simulink model "Trim_Pioneer"  (R2018a)
settings: Solver=VariableStepAuto  StartTime=0.0  StopTime=30  RelTol=1e-3  EnableMultiTasking=on
libraries: airlib x1
settings Model: Creator=MONCAYOH  LastModifiedBy=enriqueg
settings DataIOCC: SaveFormat=Array  SignalLoggingSaveFormat=ModelDataLogs  SaveOutput=off  SaveTime=off
settings OptimizationCC: BlockReduction=off  BooleanDataType=off
settings DebuggingCC: SaveWithParameterizedLinksMsg=none  UnderspecifiedInitializationDetection=Classic  MergeDetectMultiDrivingBlocksExec=none  SignalResolutionControl=TryResolveAllWithWarning  MultiTaskDSMMsg=warning  MultiTaskCondExecSysMsg=none
settings HardwareCC: TargetUnknown=on
settings ModelReferenceCC: PropagateSignalLabelsOutOfModel=off
settings CodeAppCC: StateflowObjectComments=on
settings GRTTargetCC: TargetLangStandard=C89/C90 (ANSI)  CombineOutputUpdateFcns=off  GRTInterface=on

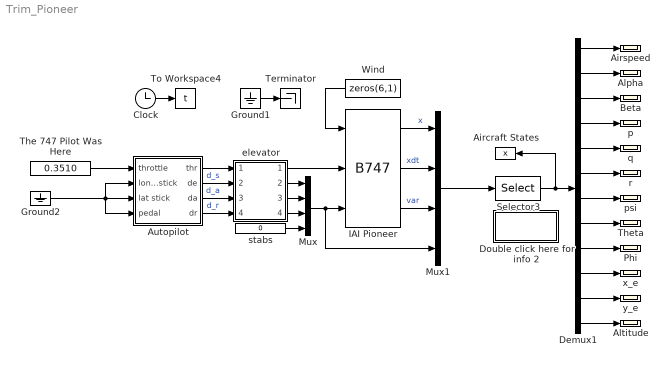
== system Trim_Pioneer ==
  " IAI Pioneer " : airlib/B747  GM1="[0.5486  5.1511  2.8261   47.2259  90.9483  111.4754   0  -6.6462  0   190.512]"  CD_wind="[0.060  0.430  0  0.0180  0]"  CL_wind="[0.385  4.78  8.05  0.401  0]"  Cm_body="[0.194  -2.12   -36.6   -1.76    0]"  CY_body="[0   -0.819    0     0    0.191    0]"  Cl_body="[0   -0.023   -0.450   0.265   -0.161  -0.00229]"  Cn_body="[0    0.109  -0.110  -0.200    0.0200  -0.0917]"  x0="[33.4389 0.1247 0   0 0 0   0 0.1247 0   0 0 150]"
  Aircraft States : ToWorkspace  VariableName=x  SampleTime=0.05
  Airspeed : Scope
  Alpha : Scope
  Altitude : Scope
  Autopilot : Subsystem
  Beta : Scope
  Clock : Clock
  Demux1 : Demux  Outputs=12
  Double click here for info 2 : Subsystem
      mask Display: disp('Output\nSignals')
  Ground1 : Ground
  Ground2 : Ground
  Mux : Mux
  Mux1 : Mux  Inputs=[12 12 12 4]
  Phi : Scope
  Selector3 : Selector  InputPortWidth=40  IndexOptions=Index vector (dialog)  Indices=1:12  OutputSizes=1
  Terminator : Terminator
  The 747 Pilot Was Here : Constant  Value=0.3510
  Theta : Scope
  To Workspace4 : ToWorkspace  VariableName=t  SampleTime=0.05
  Wind : Constant  Value=zeros(6,1)
  elevator : Subsystem
      mask Display: disp('Cable &\nactuator\ndynamics')
  p : Scope
  psi : Scope
  q : Scope
  r : Scope
  stabs : Constant  Value=0
  x_e : Scope
  y_e : Scope
  wires:
  elevator/3(deltaa) -> Mux/2
  elevator/4(deltar) -> Mux/3
  elevator/2(deltae) -> Mux/1
  Autopilot/2(de) -> elevator/2(D_elv)  "d_s"
  Autopilot/3(da) -> elevator/3(D_ail)  "d_a"
  Autopilot/4(dr) -> elevator/4(D_rud)  "d_r"
  Mux/1 -> " IAI Pioneer "/3, Mux1/4
  elevator/1(throttle) -> " IAI Pioneer "/2
  Mux1/1 -> Selector3/1
  Selector3/1 -> Demux1/1, Aircraft States/1
  Demux1/1 -> Airspeed/1
  Demux1/2 -> Alpha/1
  Demux1/3 -> Beta/1
  Demux1/4 -> p/1
  Demux1/5 -> q/1
  Demux1/6 -> r/1
  Demux1/7 -> psi/1
  Demux1/8 -> Theta/1
  Demux1/9 -> Phi/1
  Demux1/10 -> x_e/1
  Demux1/11 -> y_e/1
  Demux1/12 -> Altitude/1
  Autopilot/1(thr) -> elevator/1(D_thr)
  Clock/1 -> To Workspace4/1
  stabs/1 -> Mux/4
  Wind/1 -> " IAI Pioneer "/1
  " IAI Pioneer "/1 -> Mux1/1  "x"
  " IAI Pioneer "/2 -> Mux1/2  "xdt"
  " IAI Pioneer "/3 -> Mux1/3  "var"
  The 747 Pilot Was Here/1 -> Autopilot/1(throttle)
  Ground1/1 -> Terminator/1
  Ground2/1 -> Autopilot/4(pedal), Autopilot/3(lat stick), Autopilot/2(long stick)

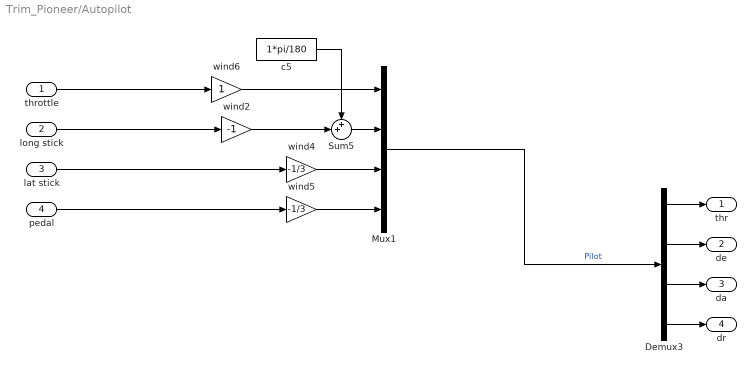
== system Trim_Pioneer/Autopilot ==
  throttle : Inport
  long stick : Inport  Port=2
  lat stick : Inport  Port=3
  pedal : Inport  Port=4
  Demux3 : Demux
  Mux1 : Mux
  Sum5 : Sum  Inputs=++|  SaturateOnIntegerOverflow=on  InputSameDT=on  OutDataTypeStr=Inherit: Same as first input
  c5 : Constant  Value=1*pi/180
  wind2 : Gain  Gain=-1  SaturateOnIntegerOverflow=on  OutDataTypeStr=Inherit: Same as input  ParamDataTypeStr=Inherit: Same as input
  wind4 : Gain  Gain=-1/3  SaturateOnIntegerOverflow=on  OutDataTypeStr=Inherit: Same as input  ParamDataTypeStr=Inherit: Same as input
  wind5 : Gain  Gain=-1/3  SaturateOnIntegerOverflow=on  OutDataTypeStr=Inherit: Same as input  ParamDataTypeStr=Inherit: Same as input
  wind6 : Gain  SaturateOnIntegerOverflow=on  OutDataTypeStr=Inherit: Same as input  ParamDataTypeStr=Inherit: Same as input
  thr : Outport
  de : Outport  Port=2
  da : Outport  Port=3
  dr : Outport  Port=4
  wires:
  long stick/1 -> wind2/1
  lat stick/1 -> wind4/1
  pedal/1 -> wind5/1
  Mux1/1 -> Demux3/1  "Pilot"
  Demux3/1 -> thr/1
  Demux3/2 -> de/1
  Demux3/3 -> da/1
  Demux3/4 -> dr/1
  wind4/1 -> Mux1/3
  wind5/1 -> Mux1/4
  throttle/1 -> wind6/1
  c5/1 -> Sum5/1
  Sum5/1 -> Mux1/2
  wind2/1 -> Sum5/2
  wind6/1 -> Mux1/1

== system Trim_Pioneer/Double click here for info 2 ==
  note: 01 v (m/s)
      | 02 alpha (rad)
      | 03 beta (rad)
      | 04 p (rad/s)
      | 05 q (rad/s)
      | 06 r  (rad/s)
      | 07 psi (rad)
      | 08 theta (rad)
      | 09 phi (rad)
      | 10 xe (m)
      | 11 ye (m)
      | 12 ze (m)
      | 13 v dot (m/s2)
      | 14 alpha dot (rad/s)
      | 15 beta dot (rad/s)
      | 16 p dot (rad/s2)
      | 17 q dot (rad/s2)
      | 18 r dot (rad/s2)
      | 19 fi dot (rad/s)
      | 20 theta dot (rad/s)
      | 21 psi dot (rad/s)
      | 22 xe dot (m/s)
      | 23 ye dot (m/s)
      | 24 ze dot (m/s)
      | 25 u dot (m/s2)
      | 26 v dot (m/s2)
      | 27 w dot (m/s2)
      | 28 pb/2v (rad)
      | 29 qc/v (rad)
      | 30 rb/v (rad)
      | 31 Ax (g)
      | 32 Ay (g)
      | 33 Az (g)
      | 34 ax (g)
      | 35 ay (g)
      | 36 az (g)
      | 37 delta elevators (rad)
      | 38 delta ailerons (rad)
      | 39 delta rudder (rad)
      | 40 delta stabs (rad)

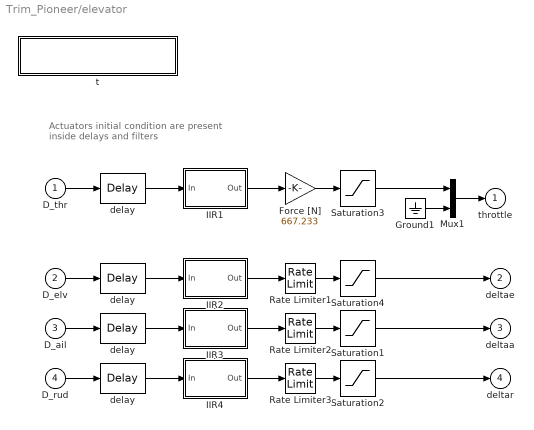
== system Trim_Pioneer/elevator ==
  note: Actuators initial condition are present
      | inside delays and filters
  D_thr : Inport
  D_elv : Inport  Port=2
  D_ail : Inport  Port=3
  D_rud : Inport  Port=4
  " delay" : TransportDelay  DelayTime=0.03  InitialOutput=-1.71374e-004
  " delay " : TransportDelay  DelayTime=0.03  InitialOutput=0.490154
  Force [N] : Gain  Gain=667.233  SaturateOnIntegerOverflow=on  OutDataTypeStr=Inherit: Same as input  ParamDataTypeStr=Inherit: Same as input
  Ground1 : Ground
  IIR1 : Subsystem  mask(Discrete Time First Order IIR){ni=1, a=4, x0=0.490154, T=0.05}
      mask prompts: ni "Number of Channels"; a "Cutoff Frequency (a)"; x0 "Initial Condition"; T "Sample Time"
      mask help:
      | Each channel has the transfer function
      |   (1-exp(-aT))/(1-exp(-aT)(z^-1)) which is a good
      |   (pz-matched) approximation of a/(s+a) if 10*a*T<pi
      mask init:
      | A=[];B=[];C=[];D=[];
      | for i=1:ni,
      | A=[A,zeros(size(A,1),1);zeros(1,size(A,2)),exp(-a*T)];
      | B=[B,zeros(size(B,1),1);zeros(1,size(B,2)),1-exp(-a*T)];
      | C=[C,zeros(size(C,1),1);zeros(1,size(C,2)),exp(-a*T)];
      | D=[D,zeros(size(D,1),1);zeros(1,size(D,2)),1-exp(-a*T)];
      | end
      mask Help:
      | <p>
      |   Each channel has the transfer function
      |   (1-exp(-aT))/(1-exp(-aT)(z^-1)) which is a good
      |   (pz-matched) approximation of a/(s+a) if 10*a*T<pi
      | </p>
      mask Display: dpoly(a,[1 a],'s')
  IIR2 : Subsystem  mask(Discrete Time First Order IIR){ni=1, a=15, x0=-1.71374e-004, T=0.05}
      mask prompts: ni "Number of Channels"; a "Cutoff Frequency (a)"; x0 "Initial Condition"; T "Sample Time"
      mask help:
      | Each channel has the transfer function
      |   (1-exp(-aT))/(1-exp(-aT)(z^-1)) which is a good
      |   (pz-matched) approximation of a/(s+a) if 10*a*T<pi
      mask init: same as Trim_Pioneer/elevator/IIR1
      mask Help:
      | <p>
      |   Each channel has the transfer function
      |   (1-exp(-aT))/(1-exp(-aT)(z^-1)) which is a good
      |   (pz-matched) approximation of a/(s+a) if 10*a*T<pi
      | </p>
      mask Display: dpoly(a,[1 a],'s')
  IIR3 : Subsystem  mask(Discrete Time First Order IIR){ni=1, a=40, x0=0, T=0.05}
      mask prompts: ni "Number of Channels"; a "Cutoff Frequency (a)"; x0 "Initial Condition"; T "Sample Time"
      mask help:
      | Each channel has the transfer function
      |   (1-exp(-aT))/(1-exp(-aT)(z^-1)) which is a good
      |   (pz-matched) approximation of a/(s+a) if 10*a*T<pi
      mask init: same as Trim_Pioneer/elevator/IIR1
      mask Help:
      | <p>
      |   Each channel has the transfer function
      |   (1-exp(-aT))/(1-exp(-aT)(z^-1)) which is a good
      |   (pz-matched) approximation of a/(s+a) if 10*a*T<pi
      | </p>
      mask Display: dpoly(a,[1 a],'s')
  IIR4 : Subsystem  mask(Discrete Time First Order IIR){ni=1, a=15, x0=0, T=0.05}
      mask prompts: ni "Number of Channels"; a "Cutoff Frequency (a)"; x0 "Initial Condition"; T "Sample Time"
      mask help:
      | Each channel has the transfer function
      |   (1-exp(-aT))/(1-exp(-aT)(z^-1)) which is a good
      |   (pz-matched) approximation of a/(s+a) if 10*a*T<pi
      mask init: same as Trim_Pioneer/elevator/IIR1
      mask Help:
      | <p>
      |   Each channel has the transfer function
      |   (1-exp(-aT))/(1-exp(-aT)(z^-1)) which is a good
      |   (pz-matched) approximation of a/(s+a) if 10*a*T<pi
      | </p>
      mask Display: dpoly(a,[1 a],'s')
  Mux1 : Mux  Inputs=[1 5]
  Rate Limiter1 : RateLimiter  RisingSlewLimit=100*pi/180  FallingSlewLimit=-100*pi/180
  Rate Limiter2 : RateLimiter  RisingSlewLimit=100*pi/180  FallingSlewLimit=-100*pi/180
  Rate Limiter3 : RateLimiter  RisingSlewLimit=100*pi/180  FallingSlewLimit=-100*pi/180
  Saturation1 : Saturate  UpperLimit=20*pi/180  LowerLimit=-20*pi/180
  Saturation2 : Saturate  UpperLimit=20*pi/180  LowerLimit=-20*pi/180
  Saturation3 : Saturate  UpperLimit=245440  LowerLimit=0
  Saturation4 : Saturate  UpperLimit=20*pi/180  LowerLimit=-20*pi/180
  delay : TransportDelay  DelayTime=0.03
  "delay " : TransportDelay  DelayTime=0.03
  t : Subsystem
      settings: OpenFcn=fdchelp actuatr
      mask Display: disp('Actuator & cable dynamics\nMarc Rauw, October 1997')
  throttle : Outport
  deltae : Outport  Port=2
  deltaa : Outport  Port=3
  deltar : Outport  Port=4
  wires:
  D_ail/1 -> delay/1
  D_elv/1 -> " delay"/1
  D_rud/1 -> "delay "/1
  IIR2/1(Out) -> Rate Limiter1/1
  Saturation4/1 -> deltae/1
  IIR3/1(Out) -> Rate Limiter2/1
  Saturation1/1 -> deltaa/1
  IIR4/1(Out) -> Rate Limiter3/1
  Saturation2/1 -> deltar/1
  Rate Limiter1/1 -> Saturation4/1
  Rate Limiter2/1 -> Saturation1/1
  Rate Limiter3/1 -> Saturation2/1
  Mux1/1 -> throttle/1
  Saturation3/1 -> Mux1/1
  Ground1/1 -> Mux1/2
  D_thr/1 -> " delay "/1
  IIR1/1(Out) -> Force [N]/1
  Force [N]/1 -> Saturation3/1
  " delay "/1 -> IIR1/1(In)
  " delay"/1 -> IIR2/1(In)
  delay/1 -> IIR3/1(In)
  "delay "/1 -> IIR4/1(In)

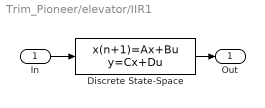
== system Trim_Pioneer/elevator/IIR1 ==
  In : Inport
  Discrete State-Space : DiscreteStateSpace  A=A  B=B  C=C  D=D  InitialCondition=x0  SampleTime=T
  Out : Outport
  wires:
  Discrete State-Space/1 -> Out/1
  In/1 -> Discrete State-Space/1

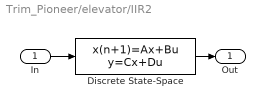
== system Trim_Pioneer/elevator/IIR2 ==
  In : Inport
  Discrete State-Space : DiscreteStateSpace  A=A  B=B  C=C  D=D  InitialCondition=x0  SampleTime=T
  Out : Outport
  wires:
  Discrete State-Space/1 -> Out/1
  In/1 -> Discrete State-Space/1

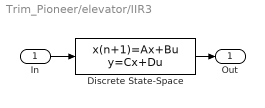
== system Trim_Pioneer/elevator/IIR3 ==
  In : Inport
  Discrete State-Space : DiscreteStateSpace  A=A  B=B  C=C  D=D  InitialCondition=x0  SampleTime=T
  Out : Outport
  wires:
  Discrete State-Space/1 -> Out/1
  In/1 -> Discrete State-Space/1

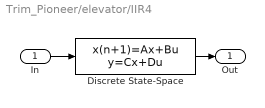
== system Trim_Pioneer/elevator/IIR4 ==
  In : Inport
  Discrete State-Space : DiscreteStateSpace  A=A  B=B  C=C  D=D  InitialCondition=x0  SampleTime=T
  Out : Outport
  wires:
  Discrete State-Space/1 -> Out/1
  In/1 -> Discrete State-Space/1

== system Trim_Pioneer/elevator/t ==
